simulink model "modelo7_circuit"  (R2023b)
settings: Solver=ode45  StartTime=0  StopTime=15  FixedStep=1  RelTol=1e-3
undefined symbols (not defined in the file): ic_values, k_values, P_max
settings Model: Creator=anruk  LastModifiedBy=anruk

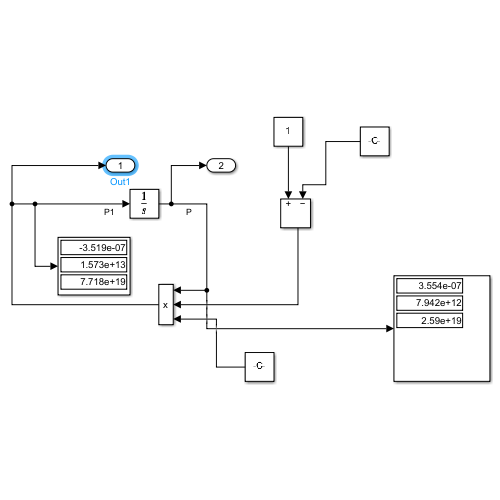
[thumbnail: Simulink's stored preview of the top-level diagram]
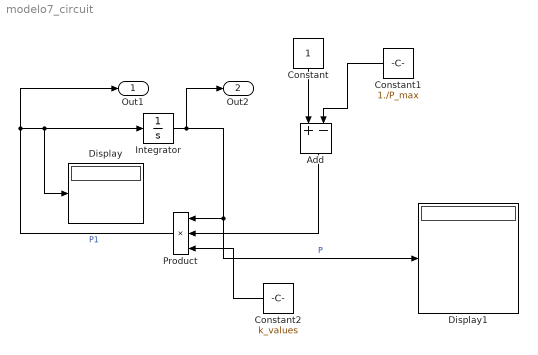
== system modelo7_circuit ==
  Add : Sum  Inputs=+-
  Constant : Constant
  Constant1 : Constant  Value=1./P_max
  Constant2 : Constant  Value=k_values
  Display : Display
  Display1 : Display
  Integrator : Integrator  InitialCondition=ic_values(:,2)
  Product : Product  Inputs=3
  Out1 : Outport
  Out2 : Outport  Port=2
  wires:
  Product/1 -> Integrator/1, Display/1, Out1/1  "P1"
  Integrator/1 -> Out2/1, Display1/1, Product/1  "P"
  Constant/1 -> Add/1
  Constant1/1 -> Add/2
  Add/1 -> Product/2
  Constant2/1 -> Product/3
